simulink model "Модель канала крена (тангажа). Симулинк"  (R2013a)
settings: Solver=ode45  StartTime=0.0  StopTime=100  RelTol=1e-3
libraries: simulink x1
settings Model: Creator=Mirag_000  LastModifiedBy=Mirag_000

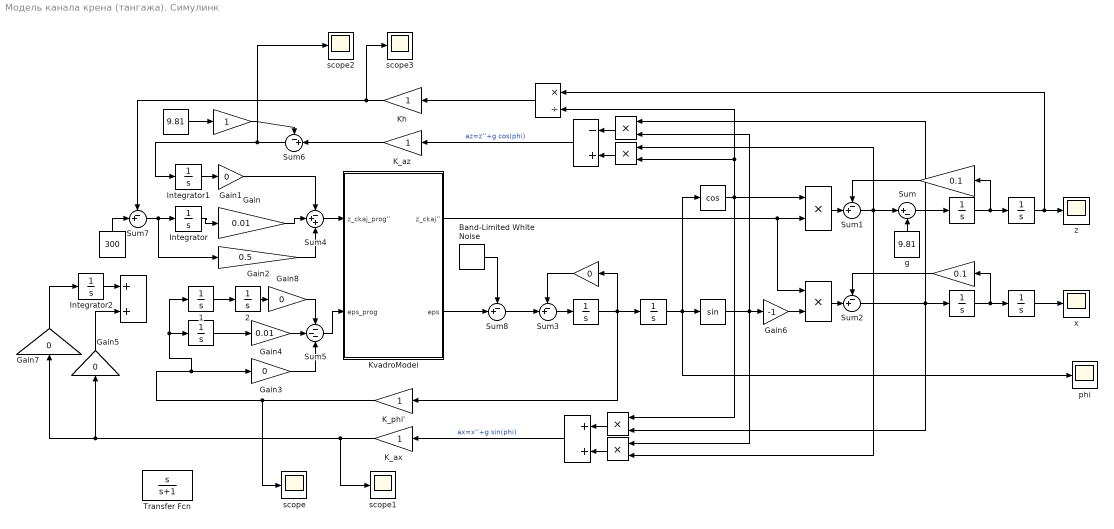
== system Модель канала крена (тангажа). Симулинк ==
  " " : Trigonometry  Operator=cos
  " " : Trigonometry
   {,,,,,,1..2} (8 alike) : Integrator
  " " : Integrator  InitialCondition=0.08
  " " : Gain  Gain=0.1
   {,,,,,} (6 alike) : Product  Inputs=**
  " " : Sum  Inputs=-+
  " " : Sum
  " " : Sum
  " " : Gain  Gain=0.1
  " " : Constant  Value=9.81
  " " : Constant  Value=300
  " " : Gain
  " " : Product  Inputs=*/
  " " : Gain  Gain=0
  Band-Limited White Noise : simulink/Sources/Band-Limited White Noise  Cov=[0]  Ts=1  seed=[23341]
  Gain : Gain  Gain=0.01
  Gain{1,3,5,7..8} (5 alike) : Gain  Gain=0
  Gain2 : Gain  Gain=0.5
  Gain4 : Gain  Gain=0.01
  Gain6 : Gain  Gain=-1
  Integrator : Integrator
  Integrator1 : Integrator
  Integrator2 : Integrator
  K_ax : Gain
  K_az : Gain
  K_phi' : Gain
  Kh : Gain
  KvadroModel : Subsystem
  Sum : Sum  Inputs=|+-
  Sum{1..3,6..8} (6 alike) : Sum  Inputs=-+|
  Sum4 : Sum  Inputs=-++
  Sum5 : Sum  Inputs=---
  Transfer Fcn : TransferFcn  Numerator=[1 0]  Denominator=[1 1]
  g : Constant  Value=9.81
  phi : Scope
      settings: TimeRange=200  YMin=-2750  YMax=250  SaveName=ScopeData2
  scope{,1..3} (4 alike) : Scope
      scope settings: TimeRange=1  YMin=-30.5  YMax=-22.5  SaveName=ScopeData3
      scope1 settings: YMin=0  YMax=4e+11  SaveName=ScopeData5
      scope2 settings: YMin=0  YMax=4e+11  SaveName=ScopeData4
      scope3 settings: YMin=0  YMax=4e+11  SaveName=ScopeData6
  x : Scope
      settings: YMin=24  YMax=34
  z : Scope
      settings: TimeRange=10  YMin=-50  YMax=300
  wires:
  " "/1 -> " "/1, phi/1, " "/1
  " "/1 -> " "/1, " "/1, " "/2, " "/2
  " "/1 -> " "/1, " "/1
  " "/1 -> " "/1, " "/1
  " "/1 -> x/1
  " "/1 -> z/1, " "/1
  " "/1 -> Sum2/2
  " "/1 -> K_az/1  "az=z''+g cos(phi)"
  " "/1 -> Gain6/1, " "/1, " "/2
  KvadroModel/1(z_ckaj'') -> " "/1, " "/2
  KvadroModel/2(eps) -> Sum8/2
  " "/1 -> Kh/1
  " "/1 -> K_phi'/1, " "/1, " "/1
  " "/1 -> Sum1/1
  " "/1 -> Sum2/1
  Sum2/1 -> " "/1, " "/2, " "/1
  g/1 -> Sum/2
  " "/1 -> Sum1/2
  " "/1 -> " "/2
  " "/1 -> " "/1
  Sum3/1 -> " "/1
  " "/1 -> Sum3/1
  " "/1 -> K_ax/1  "ax=x''+g sin(phi)"
  " "/1 -> " "/2
  " "/1 -> " "/1
  Integrator/1 -> Gain/1
  Gain/1 -> Sum4/2
  Gain2/1 -> Sum4/3
  Gain1/1 -> Sum4/1
  Sum5/1 -> KvadroModel/2(eps_prog)
  K_phi'/1 -> scope/1, " 1"/1, " "/1, Gain3/1
  Sum4/1 -> KvadroModel/1(z_ckaj_prog'')
  Integrator1/1 -> Gain1/1
  K_ax/1 -> scope1/1, Gain7/1, Gain5/1
  K_az/1 -> Sum6/2
  Sum6/1 -> scope2/1, Integrator1/1
  " "/1 -> " "/1
  " "/1 -> Sum6/1
  " "/1 -> Sum7/2
  Sum7/1 -> Gain2/1, Integrator/1
  Kh/1 -> scope3/1, Sum7/1
  Gain3/1 -> Sum5/3
  Sum/1 -> " "/1
  Sum1/1 -> " "/2, " "/1, Sum/1
  Gain4/1 -> Sum5/2
  Sum8/1 -> Sum3/2
  Gain6/1 -> " "/2
  Band-Limited White Noise/1 -> Sum8/1
  Gain5/1 -> " "/2
  Integrator2/1 -> " "/1
  Gain7/1 -> Integrator2/1
  " "/1 -> Gain4/1
  " 1"/1 -> " 2"/1
  " 2"/1 -> Gain8/1
  Gain8/1 -> Sum5/1

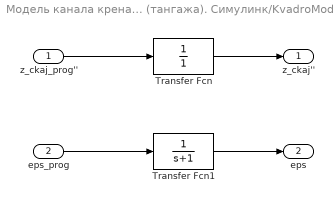
== system Модель канала крена (тангажа). Симулинк/KvadroModel ==
  z_ckaj_prog'' : Inport
  eps_prog : Inport  Port=2
  Transfer Fcn : TransferFcn  Denominator=[0 1]
  Transfer Fcn1 : TransferFcn  Denominator=[1 1]
  z_ckaj'' : Outport
  eps : Outport  Port=2
  wires:
  z_ckaj_prog''/1 -> Transfer Fcn/1
  eps_prog/1 -> Transfer Fcn1/1
  Transfer Fcn/1 -> z_ckaj''/1
  Transfer Fcn1/1 -> eps/1
